simulink library "Lib_JARVISPH2_deVCU_Mem"  (R2019b)
settings: Solver=ode45  StartTime=0.0  StopTime=10.0  RelTol=1e-3  EnableMultiTasking=on
settings Model: Creator=kmansour  LastModifiedBy=User
settings DataIOCC: LimitDataPoints=on  SaveFormat=Array  ReturnWorkspaceOutputs=off
settings OptimizationCC: LifeSpan=inf
settings DebuggingCC: AllowSymbolicDim=off  SFUnexpectedBacktrackingDiag=warning  SFNoUnconditionalDefaultTransitionDiag=warning  SFExecutionAtInitializationDiag=none  ArithmeticOperatorsInVariantConditions=warning
settings HardwareCC: ProdBitPerPointer=32  ProdBitPerSizeT=32  ProdBitPerPtrDiffT=32  ProdLargestAtomicFloat=None  ProdIntDivRoundTo=Undefined  ProdEndianess=Unspecified  ProdWordSize=32  ProdHWDeviceType=32-bit Generic
settings ModelReferenceCC: PropagateSignalLabelsOutOfModel=off
settings SFSimCC: SimUseLocalCustomCode=off  CustomCodeUndefinedFunction=UseInterfaceOnly
settings RTWCC: RTWUseLocalCustomCode=off
settings CodeAppCC: StateflowObjectComments=on
settings GRTTargetCC: TargetLangStandard=C89/C90 (ANSI)  GeneratePreprocessorConditionals=Disable all
settings ConfigComp: CovMetricSettings=dw  CovHtmlReporting=on  CovSaveCumulativeToWorkspaceVar=on  CovSaveSingleToWorkspaceVar=on  CovExternalEMLEnable=off

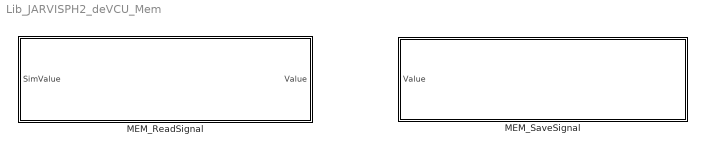
== system Lib_JARVISPH2_deVCU_Mem ==
  MEM_ReadSignal : Subsystem  TreatAsAtomicUnit=on  mask{PARAM_ID=ECU_MEM_INT_PREVIOUS_ENERGY_CONSUMPTION}
      mask prompts: PARAM_ID "Choose a Signal"
      mask TypeOptions PARAM_ID: ECU_MEM_INT_PREVIOUS_ENERGY_CONSUMPTION | ECU_MEM_INT_EEPROM_BOOTNUMBER | ECU_MEM_INT_CLB_NONAME_2 | ECU_MEM_INT_CLB_NONAME_3 | ECU_MEM_INT_CLB_NONAME_4 | ECU_MEM_INT_CLB_NONAME_5 | ECU_MEM_INT_CLB_NONAME_6 | ECU_MEM_INT_CLB_NONAME_7 | ECU_MEM_INT_CLB_NONAME_8
      mask Display:
      | image(imread('devcu_final.png'),'top-left');
      | color('black');
      | port_label('input', 1, 'SimValue');
      | port_label('output', 1, 'Value');
      | 
      | strCell =get_param(gcb, 'MaskValues');
      | strCell = strtrim(strCell);
      | str = strCell{1};
      | str = strrep(str, '_', '\_');
      | disp(str, 'texmode', 'on');
  MEM_SaveSignal : Subsystem  TreatAsAtomicUnit=on  mask{PARAM_ID=ECU_MEM_INT_PREVIOUS_ENERGY_CONSUMPTION}
      mask prompts: PARAM_ID "Choose a Signal"
      mask TypeOptions PARAM_ID: ECU_MEM_INT_PREVIOUS_ENERGY_CONSUMPTION | ECU_MEM_INT_EEPROM_BOOTNUMBER | ECU_MEM_INT_CLB_NONAME_2 | ECU_MEM_INT_CLB_NONAME_3 | ECU_MEM_INT_CLB_NONAME_4 | ECU_MEM_INT_CLB_NONAME_5 | ECU_MEM_INT_CLB_NONAME_6 | ECU_MEM_INT_CLB_NONAME_7 | ECU_MEM_INT_CLB_NONAME_8
      mask Display:
      | image(imread('devcu_final.png'),'top-right');
      | color('black');
      | port_label('input', 1, 'Value');
      | 
      | strCell =get_param(gcb, 'MaskValues');
      | strCell = strtrim(strCell);
      | str = strCell{1};
      | str = strrep(str, '_', '\_');
      | disp(str, 'texmode', 'on');

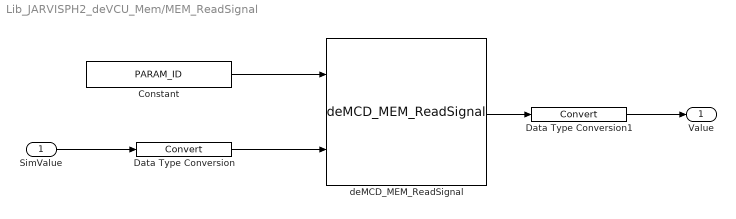
== system Lib_JARVISPH2_deVCU_Mem/MEM_ReadSignal ==
  SimValue : Inport
  Constant : Constant  Value=PARAM_ID
  Data Type Conversion : DataTypeConversion
  Data Type Conversion1 : DataTypeConversion
  deMCD_MEM_ReadSignal : S-Function  FunctionName=deMCD_MEM_ReadSignal  SFunctionDeploymentMode=off  EnableBusSupport=off
      mask Display:
      | image(imread('logo_deMCD_white_background.png'),'center');
      | color('black');
      | port_label('input', 1, 'ID');
      | port_label('input', 2, 'SimValue');
      | port_label('output', 1, 'Value');
  Value : Outport
  wires:
  deMCD_MEM_ReadSignal/1 -> Data Type Conversion1/1
  Constant/1 -> deMCD_MEM_ReadSignal/1
  Data Type Conversion/1 -> deMCD_MEM_ReadSignal/2
  Data Type Conversion1/1 -> Value/1
  SimValue/1 -> Data Type Conversion/1

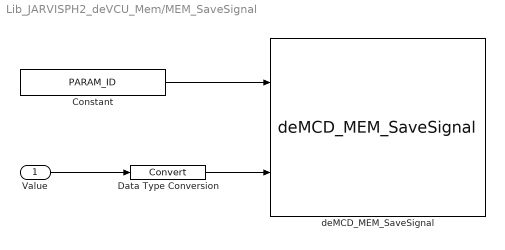
== system Lib_JARVISPH2_deVCU_Mem/MEM_SaveSignal ==
  Value : Inport
  Constant : Constant  Value=PARAM_ID
  Data Type Conversion : DataTypeConversion
  deMCD_MEM_SaveSignal : S-Function  FunctionName=deMCD_MEM_SaveSignal  SFunctionDeploymentMode=off  EnableBusSupport=off
      mask Display:
      | image(imread('logo_deMCD_white_background.png'),'center');
      | color('black');
      | port_label('input', 1, 'ID');
      | port_label('input', 2, 'Value');
  wires:
  Constant/1 -> deMCD_MEM_SaveSignal/1
  Value/1 -> Data Type Conversion/1
  Data Type Conversion/1 -> deMCD_MEM_SaveSignal/2
